simulink model "Vaccum"  (R2022b)
settings: Solver=VariableStepAuto  StartTime=0.0  StopTime=10.0  RelTol=1e-3
settings Model: Creator=11  LastModifiedBy=11

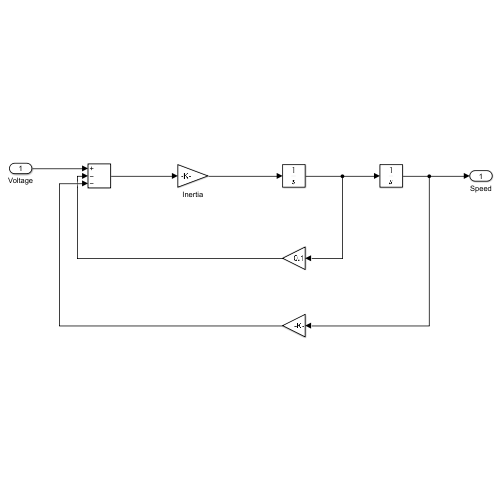
[thumbnail: Simulink's stored preview of the top-level diagram]
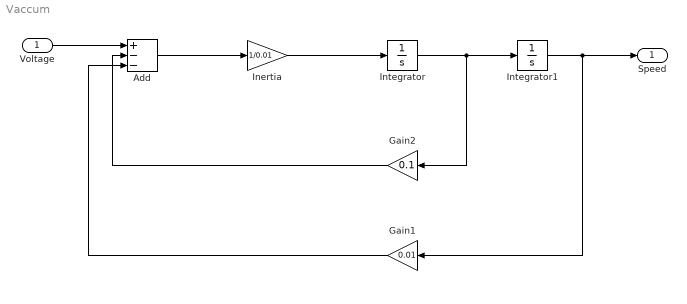
== system Vaccum ==
  Voltage : Inport
  Add : Sum  Inputs=+--
  Gain1 : Gain  Gain=0.01
  Gain2 : Gain  Gain=0.1
  Inertia : Gain  Gain=1/0.01
  Integrator : Integrator
  Integrator1 : Integrator
  Speed : Outport
  wires:
  Voltage/1 -> Add/1
  Add/1 -> Inertia/1
  Inertia/1 -> Integrator/1
  Integrator/1 -> Gain2/1, Integrator1/1
  Integrator1/1 -> Gain1/1, Speed/1
  Gain2/1 -> Add/2
  Gain1/1 -> Add/3
